simulink model "MultirotorSimPx4v1_8ContAttOnly"  (R2018b)
settings: Solver=VariableStepAuto  StartTime=0.0  StopTime=Simulation.T_END  MaxStep=Simulation.TS_MAX  RelTol=1e-3  EnableMultiTasking=on
PreLoadFcn:
  | % InitializeParameters;
undefined symbols (not defined in the file): Initial, Uav, Wind
libraries: simulink_extras x4, QuaternionLibrary x3
settings Model: Creator=jban039  LastModifiedBy=jban039
settings DataIOCC: Decimation=10  ExternalInput=getinputstruct(report10)  InitialState=getstatestruct(op)  LoadInitialState=on  SignalLogging=off  ReturnWorkspaceOutputs=on  OutputOption=SpecifiedOutputTimes  OutputTimes=Simulation.T_OUT
settings OptimizationCC: LifeSpan=inf
settings DebuggingCC: ReadBeforeWriteMsg=DisableAll  WriteAfterWriteMsg=DisableAll  WriteAfterReadMsg=DisableAll  MultiTaskDSMMsg=none  UnconnectedLineMsg=none  AllowSymbolicDim=off  SFUnexpectedBacktrackingDiag=warning  SFNoUnconditionalDefaultTransitionDiag=warning  SFExecutionAtInitializationDiag=none  UnderSpecifiedDimensionMsg=warning
settings ModelReferenceCC: UpdateModelReferenceTargets=IfOutOfDate  ModelReferenceMinAlgLoopOccurrences=on  PropagateSignalLabelsOutOfModel=off
settings SFSimCC: SFSimEcho=off  SimUseLocalCustomCode=off
settings RTWCC: RTWUseLocalCustomCode=off
settings CodeAppCC: StateflowObjectComments=on
settings GRTTargetCC: TargetLangStandard=C89/C90 (ANSI)
settings ConfigComp: CovMetricSettings=dw  CovHtmlReporting=on  CovSaveCumulativeToWorkspaceVar=on  CovSaveSingleToWorkspaceVar=on  CovExternalEMLEnable=off

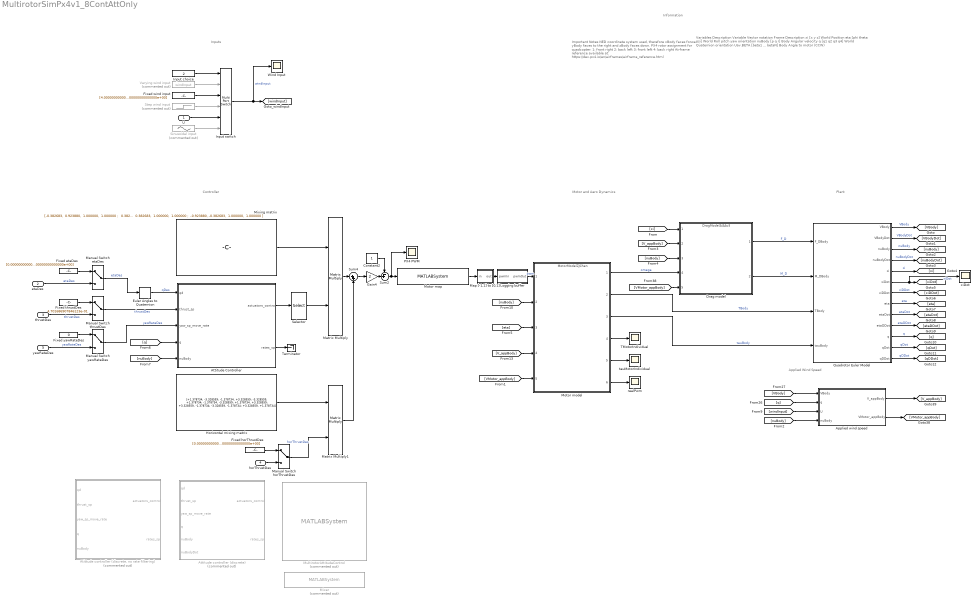
== system MultirotorSimPx4v1_8ContAttOnly ==
  note: Important Notes
      |
      | NED coordinate system used, therefore xBody faces forward, yBody faces to the right and zBody faces down.
      | PX4 rotor assignment for quadcopter:
      | 1: front right
      | 2: back left
      | 3: front left
      | 4: back right
      | Airframe reference available at:
      | https://dev.px4.io/en/airframes/airframe_reference.html
  note: Variables Description
      |
      | Variable
      | Vector notation
      | Frame
      | Description
      |
      | xi
      | [x y z]
      | World
      | Position
      |
      | eta
      | [phi theta psi]
      | World
      | Roll pitch yaw orientation
      |
      | nuBody
      | [p q r]
      | Body
      | Angular velocity
      |
      | q
      | [q1 q2 q3 q4]
      | World
      | Quaternion orientation
      |
      | Uav.BETA
      | [beta1 ... betaN]
      | Body
      | Angle to motor (CCW)
  note: Inputs
  note: Plant
  note: Motor and Aero Dynamics
  note: Information
  note: Controller
  note: Applied Wind Speed
  U : Inport  PortDimensions=3
  etaDes : Inport  Port=2  PortDimensions=[3,1]
  thrustDes : Inport  Port=3  PortDimensions=1
  horThrustDes : Inport  Port=4  PortDimensions=2
  yawRateDes : Inport  Port=5  PortDimensions=1
  Applied wind speed : Subsystem
  "Atittude controller (discrete, no rate filtering)" : Subsystem  Commented=on
  Attitude Controller : Subsystem
      mask Display: fprintf('MC_ATT_CONTROL\n\nCONTINUOUS')
  Attitude controller (discrete) : Subsystem  Commented=on
  Constant2 : Constant
  Drag model : ModelReference  ModelNameDialog=DragModelAIAAv3  SimulationMode=Normal  ModelReferenceVersion=1.368
  Euler Angles to Quaternion : QuaternionLibrary/Euler Angles to Quaternion
  Fixed etaDes : Constant  Value=[0.000000000000000e+00;-7.819550824259679e-02;0.000000000000000e+00]
  Fixed horThrustDes : Constant  Value=[0.000000000000000e+00;0.000000000000000e+00]
  Fixed thrustDes : Constant  Value=4.701686907846123e-01
  Fixed wind input : Constant  Value=[4.000000000000000e+00;0.000000000000000e+00;0.000000000000000e+00]
  Fixed yawRateDes : Constant  Value=0
  Gain4 : Gain  Gain=2
  Horizontal mixing matrix : Constant  Value=|
      | [+1.378734, -3.328559;
      |  -1.378734, +3.328559;
      |  -3.328559, +1.378734;
      |  -1.378734, -3.328559;
      |  +1.378734, +3.328559;
      |  +3.328559, -1.378734;
      |  -3.328559, -1.378734;
      |  +3.328559, +1.378734]
  Input choice : Constant  Value=2
  Input switch : MultiPortSwitch  Inputs=5
  Logging buffer : Subsystem
  Manual Switch etaDes : ManualSwitch
  Manual Switch horThrustDes : ManualSwitch
  Manual Switch thrustDes : ManualSwitch
  Manual Switch yawRateDes : ManualSwitch
  Map [-1,1] to [0,1] : Subsystem
  Matrix Multiply : Product  Multiplication=Matrix(*)
  Matrix Multiply1 : Product  Multiplication=Matrix(*)
  Mixer : MATLABSystem  Commented=on  SCDEnableBlockLinearizationSpecification=on  System=MultirotorMixer  airframeConfig=5  useHorThrust=0  outputSatStatus=0  SimulateUsing=Interpreted execution
      mask Type: MultirotorMixer
      mask Display:
      | disp(['MULTIROTOR' char(10) 'MIXER' char(10) 'octa_x']);
      | port_label('input',1,'actuatorsControl');
      | port_label('output',1,'px4PWM');
  Mixing matrix : Constant  Value=|
      | [-0.382683,  0.923880,  1.000000,  1.000000 ;
      |   0.382683, -0.923880,  1.000000,  1.000000 ;
      |  -0.923880,  0.382683, -1.000000,  1.000000 ;
      |  -0.382683, -0.923880, -1.000000,  1.000000 ;
      |   0.382683,  0.923880, -1.000000,  1.000000 ;
      |   0.923880, -0.382683, -1.000000,  1.000000 ;
      |   0.923880,  0.382683,  1.000000,  1.000000 ;
      |  -0.923880, -0.382683,  1.000000,  1.000000 ]
  Motor map : MATLABSystem  System=MotorMap  airframeConfig=5  SimulateUsing=Code generation
      mask Type: MotorMap
      mask Display:
      | disp(['MOTOR' char(10) 'MAP' char(10) 'octa_x']);
      | port_label('input',1,'px4PWM');
      | port_label('output',1,'simPWM');
  Motor model : ModelReference  ModelNameDialog=MotorModelZJChen  SimulationMode=Normal  ModelReferenceVersion=1.422
  MultirotorAttitudeControl : MATLABSystem  Commented=on  System=MulticopterAttitudeControl  acro_expo_rp=0.69  acro_expo_y=0.69  acro_pitch_max=720  acro_roll_max=720  acro_superexpo_rp=0.7  acro_superexpo_y=0.7  acro_yaw_max=540  airmode=0  d_term_cutoff_freq=30  pitch_rate_d=0.003  pitch_rate_ff=0  pitch_rate_i=0.05  pitch_rate_max=220  pitch_rate_p=0.15  pitch_p=6.5  pitch_rate_integ_lim=0.3  rattitude_thres=0.8  roll_rate_d=0.003  roll_rate_ff=0  roll_rate_i=0.05  roll_rate_max=220  roll_rate_p=0.15  roll_p=6.5  roll_rate_integ_lim=0.3  tpa_breakpoint_d=1  tpa_breakpoint_i=1  tpa_breakpoint_p=1  tpa_rate_d=0  tpa_rate_i=0  tpa_rate_p=0  yaw_rate_d=0  yaw_rate_ff=0  yaw_rate_i=0.1  yaw_rate_max=200  yaw_rate_p=0.2  yaw_auto_max=45  yaw_p=2.8  yaw_rate_integ_lim=0.3  man_throttle_min=0.08  man_tilt_max_deg=35  yaw_rate_scaling=200  throttle_hover=0.5  throttle_max=1  board_rotation_param=0  board_offset_x=0  board_offset_y=0  board_offset_z=0  bat_scale_en=0  throttle_curve=0  vehicle_status_is_rotary_wing=1  vehicle_status_is_vtol=0  loop_update_rate_hz=250  simple_mode=1  output_rates=0  SimulateUsing=Code generation
      mask Type: MulticopterAttitudeControl
      mask Display:
      | disp(['MulticopterAttitudeControl' char(10) '' char(10) 'v1.82']);
      | port_label('input',1,'qDes');
      | port_label('input',2,'thrustDes');
      | port_label('input',3,'yawRateDes');
      | port_label('input',4,'qMeasured');
      | port_label('input',5,'nuBody');
      | port_label('output',1,'actuatorsControl');
  PX4 PWM : Scope
  Quadrotor Euler Model : Subsystem
  Selector : Selector  InputPortWidth=8  IndexOptions=Index vector (dialog)  Indices=[1:4]  OutputSizes=1
  Sinusoidal input : Sin  Commented=on  Amplitude=Wind.Ampl  Bias=Wind.Bias  Frequency=Wind.Freq  SampleTime=0
  Step wind input : Step  Commented=on  Time=5  Before=[3 0 0]'  After=[5 0 0]'  SampleTime=0
  Sum2 : Sum  Inputs=-+|
  Sum4 : Sum  Inputs=|++
  TMotorIndividual : Scope
  Terminator : Terminator
  Varying wind input : FromWorkspace  Commented=on  VariableName=windInput  SampleTime=0
  Wind Input : Scope
  realPwm : Scope
  tauMotorIndividual : Scope
  xiDot : Scope
  wires:
  Motor model/1 -> Drag model/4  "omega"
  Motor model/2 -> Quadrotor Euler Model/3(TBody)  "TBody"
  Drag model/2 -> Quadrotor Euler Model/2(M_DBody)  "M_D"
  Quadrotor Euler Model/1(VBody) -> [VBody]  "VBody"
  Quadrotor Euler Model/2(VBodyDot) -> [VBodyDot]  "VBodyDot"
  Quadrotor Euler Model/3(nuBody) -> [nuBody]  "nuBody"
  Quadrotor Euler Model/4(nuBodyDot) -> [nuBodyDot]  "nuBodyDot"
  Quadrotor Euler Model/5(xi) -> [xi]  "xi"
  Quadrotor Euler Model/6(xiDot) -> xiDot/1, [xiDot]  "xiDot"
  Quadrotor Euler Model/7(xiDDot) -> [xiDDot]  "xiDDot"
  Quadrotor Euler Model/8(eta) -> [eta]  "eta"
  Quadrotor Euler Model/9(etaDot) -> [etaDot]  "etaDot"
  Quadrotor Euler Model/10(etaDDot) -> [etaDDot]  "etaDDot"
  [V_appBody] -> Drag model/2
  [nuBody] -> Motor model/2
  Quadrotor Euler Model/11(q) -> [q]  "q"
  Quadrotor Euler Model/12(qDot) -> [qDot]  "qDot"
  Quadrotor Euler Model/13(qDDot) -> [qDDot]  "qDDot"
  Drag model/1 -> Quadrotor Euler Model/1(F_DBody)  "F_D"
  Logging buffer/1(pwmOut) -> Motor model/1  "pwm"
  Sum2/1 -> PX4 PWM/1, Motor map/1
  [nuBody] -> Drag model/3
  [eta] -> Motor model/3
  [V_appBody] -> Motor model/4
  Motor model/4 -> TMotorIndividual/1
  Motor model/5 -> tauMotorIndividual/1
  [xi] -> Drag model/1
  [VMotor_appBody] -> Motor model/5
  [VMotor_appBody] -> Drag model/5
  Euler Angles to Quaternion/1 -> Attitude Controller/1(qd)  "qDes"
  Manual Switch thrustDes/1 -> Attitude Controller/2(thrust_sp)  "thrustDes"
  Manual Switch yawRateDes/1 -> Attitude Controller/3(yaw_sp_move_rate)  "yawRateDes"
  Motor model/3 -> Quadrotor Euler Model/4(tauBody)  "tauBody"
  [VBody] -> Applied wind speed/1(VBody)
  [q] -> Applied wind speed/2(q)
  [windInput] -> Applied wind speed/3(U)
  Applied wind speed/1(V_appBody) -> [V_appBody]
  Applied wind speed/2(VMotor_appBody) -> [VMotor_appBody]
  [nuBody] -> Applied wind speed/4(nuBody)
  Motor model/6 -> realPwm/1
  Motor map/1 -> Map [-1,1] to [0,1]/1(in)
  Map [-1,1] to [0,1]/1(out) -> Logging buffer/1(pwmIn)
  Selector/1 -> Matrix Multiply/2
  Manual Switch etaDes/1 -> Euler Angles to Quaternion/1  "etaDes"
  Attitude Controller/1(actuators_control) -> Selector/1
  Gain4/1 -> Sum2/2
  Constant2/1 -> Sum2/1
  Matrix Multiply/1 -> Sum4/1
  Matrix Multiply1/1 -> Sum4/2
  Manual Switch horThrustDes/1 -> Matrix Multiply1/2  "horThrustDes"
  Attitude Controller/2(rates_sp) -> Terminator/1
  Mixing matrix/1 -> Matrix Multiply/1
  Horizontal mixing matrix/1 -> Matrix Multiply1/1
  Sum4/1 -> Gain4/1
  [q] -> Attitude Controller/4(q)
  [nuBody] -> Attitude Controller/5(nuBody)
  Sinusoidal input/1 -> Input switch/6
  U/1 -> Input switch/5
  Input choice/1 -> Input switch/1
  Step wind input/1 -> Input switch/4
  Input switch/1 -> [windInput], Wind Input/1  "windInput"
  Fixed wind input/1 -> Input switch/3
  Varying wind input/1 -> Input switch/2
  Fixed horThrustDes/1 -> Manual Switch horThrustDes/1
  Fixed thrustDes/1 -> Manual Switch thrustDes/1
  Fixed etaDes/1 -> Manual Switch etaDes/1
  etaDes/1 -> Manual Switch etaDes/2  "etaDes"
  thrustDes/1 -> Manual Switch thrustDes/2  "thrustDes"
  yawRateDes/1 -> Manual Switch yawRateDes/2  "yawRateDes"
  horThrustDes/1 -> Manual Switch horThrustDes/2
  Fixed yawRateDes/1 -> Manual Switch yawRateDes/1

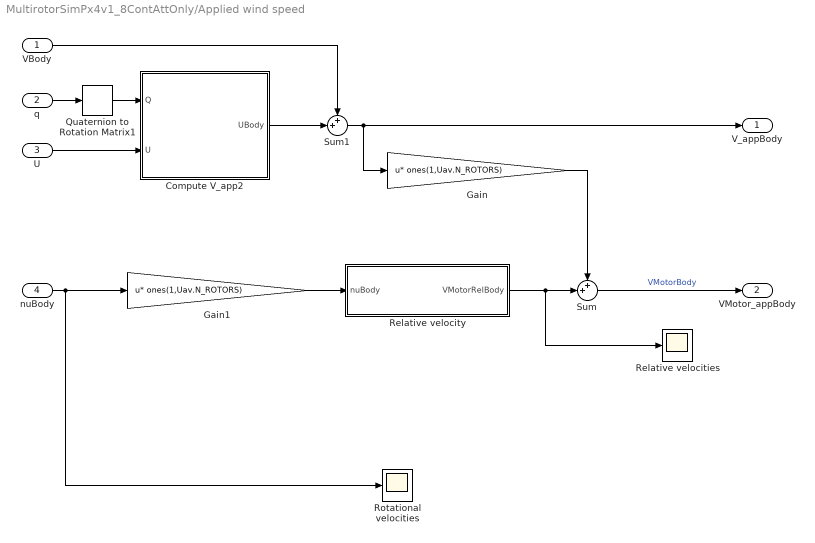
== system MultirotorSimPx4v1_8ContAttOnly/Applied wind speed ==
  VBody : Inport  Unit=m/s
  q : Inport  Port=2
  U : Inport  Port=3  Unit=m/s
  nuBody : Inport  Port=4  Unit=rad/s
  Compute V_app2 : MATLAB Function  TreatAsAtomicUnit=on
  Gain : Gain  Gain=ones(1,Uav.N_ROTORS)  Multiplication=Matrix(u*K)
  Gain1 : Gain  Gain=ones(1,Uav.N_ROTORS)  Multiplication=Matrix(u*K)
  Quaternion to Rotation Matrix1 : QuaternionLibrary/Quaternion to Rotation Matrix
  Relative velocities : Scope
  Relative velocity : MATLAB Function  TreatAsAtomicUnit=on
  Rotational velocities : Scope
  Sum : Sum  Inputs=++|
  Sum1 : Sum  Inputs=++|
  V_appBody : Outport  Unit=m/s
  VMotor_appBody : Outport  Port=2  Unit=m/s  PortDimensions=[3,Uav.N_ROTORS]
  wires:
  U/1 -> Compute V_app2/2(U)
  Sum/1 -> VMotor_appBody/1  "VMotorBody"
  Quaternion to Rotation Matrix1/1 -> Compute V_app2/1(Q)
  nuBody/1 -> Gain1/1, Rotational velocities/1
  Gain/1 -> Sum/1
  VBody/1 -> Sum1/1
  q/1 -> Quaternion to Rotation Matrix1/1
  Relative velocity/1(VMotorRelBody) -> Relative velocities/1, Sum/2
  Compute V_app2/1(UBody) -> Sum1/2
  Sum1/1 -> Gain/1, V_appBody/1
  Gain1/1 -> Relative velocity/1(nuBody)

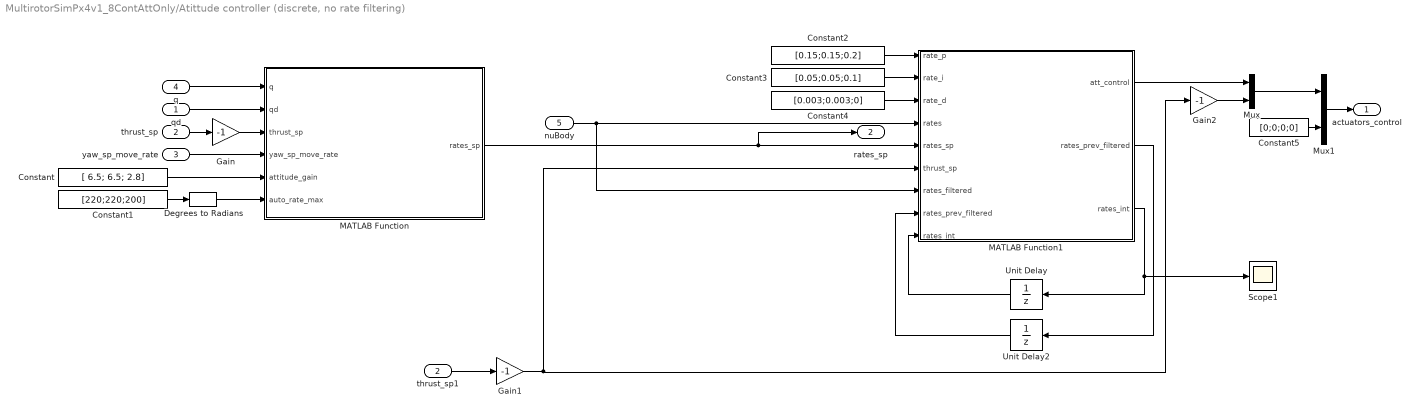
== system MultirotorSimPx4v1_8ContAttOnly/Atittude controller (discrete, no rate filtering) ==
  qd : Inport
  thrust_sp : Inport  Port=2
  yaw_sp_move_rate : Inport  Port=3
  q : Inport  Port=4
  nuBody : Inport  Port=5
  Constant : Constant  Value=[ 6.5; 6.5; 2.8]
  Constant1 : Constant  Value=[220;220;200]
  Constant2 : Constant  Value=[0.15;0.15;0.2]
  Constant3 : Constant  Value=[0.05;0.05;0.1]
  Constant4 : Constant  Value=[0.003;0.003;0]
  Constant5 : Constant  Value=[0;0;0;0]
  Degrees to Radians : simulink_extras/Transformations/Degrees to Radians
  Gain : Gain  Gain=-1
  Gain1 : Gain  Gain=-1
  Gain2 : Gain  Gain=-1
  MATLAB Function : MATLAB Function  TreatAsAtomicUnit=on  SystemSampleTime=1/250
  MATLAB Function1 : MATLAB Function  TreatAsAtomicUnit=on  SystemSampleTime=1/250
  Mux : Mux  Inputs=2
  Mux1 : Mux  Inputs=2
  Scope1 : Scope
  Unit Delay : UnitDelay  SampleTime=1/250  StateName=rates_int
  Unit Delay2 : UnitDelay  SampleTime=1/250  StateName=rates_prev_filtered
  thrust_sp1 : InportShadow  Port=2
  actuators_control : Outport
  rates_sp : Outport  Port=2
  wires:
  qd/1 -> MATLAB Function/2(qd)
  q/1 -> MATLAB Function/1(q)
  Constant/1 -> MATLAB Function/5(attitude_gain)
  Constant1/1 -> Degrees to Radians/1
  Degrees to Radians/1 -> MATLAB Function/6(auto_rate_max)
  yaw_sp_move_rate/1 -> MATLAB Function/4(yaw_sp_move_rate)
  Constant4/1 -> MATLAB Function1/3(rate_d)
  Constant3/1 -> MATLAB Function1/2(rate_i)
  Constant2/1 -> MATLAB Function1/1(rate_p)
  MATLAB Function1/1(att_control) -> Mux/1
  nuBody/1 -> MATLAB Function1/7(rates_filtered), MATLAB Function1/4(rates)
  Unit Delay/1 -> MATLAB Function1/9("rates_int ")
  MATLAB Function1/3(rates_int) -> Unit Delay/1, Scope1/1
  Mux/1 -> Mux1/1
  Unit Delay2/1 -> MATLAB Function1/8("rates_prev_filtered ")
  MATLAB Function1/2(rates_prev_filtered) -> Unit Delay2/1
  thrust_sp1/1 -> Gain1/1
  Constant5/1 -> Mux1/2
  Mux1/1 -> actuators_control/1
  thrust_sp/1 -> Gain/1
  MATLAB Function/1(rates_sp) -> MATLAB Function1/5(rates_sp), rates_sp/1
  Gain/1 -> MATLAB Function/3(thrust_sp)
  Gain1/1 -> Gain2/1, MATLAB Function1/6(thrust_sp)
  Gain2/1 -> Mux/2

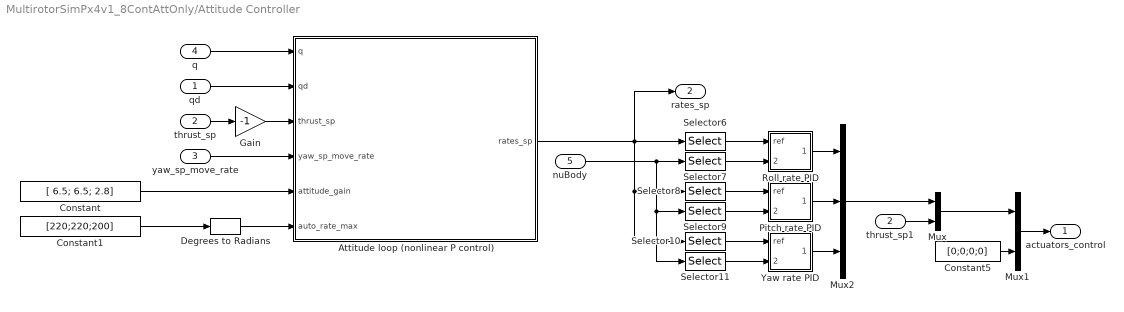
== system MultirotorSimPx4v1_8ContAttOnly/Attitude Controller ==
  qd : Inport
  thrust_sp : Inport  Port=2  PortDimensions=1
  yaw_sp_move_rate : Inport  Port=3
  q : Inport  Port=4
  nuBody : Inport  Port=5
  Attitude loop (nonlinear P control) : MATLAB Function  TreatAsAtomicUnit=on
  Constant : Constant  Value=[ 6.5; 6.5; 2.8]
  Constant1 : Constant  Value=[220;220;200]
  Constant5 : Constant  Value=[0;0;0;0]
  Degrees to Radians : simulink_extras/Transformations/Degrees to Radians
  Gain : Gain  Gain=-1
  Mux : Mux  Inputs=2
  Mux1 : Mux  Inputs=2
  Mux2 : Mux  Inputs=3
  Pitch rate PID : Subsystem  mask{PID_P=0.15, PID_I=0.05, PID_D=0.003, PID_FC=30, PID_I_STATENAME='AttRatePID_I_pitch', PID_D_STATENAME='AttRatePID_D_pitch'}
      mask prompts: PID_P "P gain"; PID_I "I gain"; PID_D "D gain"; PID_FC "D filter cutoff (Hz)"; PID_I_STATENAME "Integartor state name"; PID_D_STATENAME "D filter state name"
      mask DialogControl DescGroupVar Prompt: PID Controller with Second Order Derivative Filter
      mask DialogControl DescTextVar Prompt: The derivative gain is applied on the derivative of y rather than that of the error (r-y).
      mask Display:
      | disp('PID(s)')
      | port_label('input', 1, 'r')
      | port_label('input', 2, 'y')
      | text(1,0,'2^{nd}','horizontalAlignment','right','interpreter','tex','verticalAlignment','bottom')
  Roll rate PID : Subsystem  mask{PID_P=0.15, PID_I=0.05, PID_D=0.003, PID_FC=30, PID_I_STATENAME='AttRatePID_I_roll', PID_D_STATENAME='AttRatePID_D_roll'}
      mask prompts: PID_P "P gain"; PID_I "I gain"; PID_D "D gain"; PID_FC "D filter cutoff (Hz)"; PID_I_STATENAME "Integartor state name"; PID_D_STATENAME "D filter state name"
      mask DialogControl DescGroupVar Prompt: PID Controller with Second Order Derivative Filter
      mask DialogControl DescTextVar Prompt: The derivative gain is applied on the derivative of y rather than that of the error (r-y).
      mask Display:
      | disp('PID(s)')
      | port_label('input', 1, 'r')
      | port_label('input', 2, 'y')
      | text(1,0,'2^{nd}','horizontalAlignment','right','interpreter','tex','verticalAlignment','bottom')
  Selector10 : Selector  InputPortWidth=3  IndexOptions=Index vector (dialog)  Indices=3  OutputSizes=1
  Selector11 : Selector  InputPortWidth=3  IndexOptions=Index vector (dialog)  Indices=3  OutputSizes=1
  Selector6 : Selector  InputPortWidth=3  IndexOptions=Index vector (dialog)  Indices=1  OutputSizes=1
  Selector7 : Selector  InputPortWidth=3  IndexOptions=Index vector (dialog)  Indices=1  OutputSizes=1
  Selector8 : Selector  InputPortWidth=3  IndexOptions=Index vector (dialog)  Indices=2  OutputSizes=1
  Selector9 : Selector  InputPortWidth=3  IndexOptions=Index vector (dialog)  Indices=2  OutputSizes=1
  Yaw rate PID : Subsystem  mask{PID_P=0.2, PID_I=0.1, PID_D=0, PID_FC=30, PID_I_STATENAME='AttRatePID_I_yaw', PID_D_STATENAME='AttRatePID_D_yaw'}
      mask prompts: PID_P "P gain"; PID_I "I gain"; PID_D "D gain"; PID_FC "D filter cutoff (Hz)"; PID_I_STATENAME "Integartor state name"; PID_D_STATENAME "D filter state name"
      mask DialogControl DescGroupVar Prompt: PID Controller with Second Order Derivative Filter
      mask DialogControl DescTextVar Prompt: The derivative gain is applied on the derivative of y rather than that of the error (r-y).
      mask Display:
      | disp('PID(s)')
      | port_label('input', 1, 'r')
      | port_label('input', 2, 'y')
      | text(1,0,'2^{nd}','horizontalAlignment','right','interpreter','tex','verticalAlignment','bottom')
  thrust_sp1 : InportShadow  Port=2  PortDimensions=1
  actuators_control : Outport  PortDimensions=8
  rates_sp : Outport  Port=2
  wires:
  nuBody/1 -> Selector7/1, Selector9/1, Selector11/1
  Selector9/1 -> Pitch rate PID/2(meas)
  Selector11/1 -> Yaw rate PID/2(meas)
  Selector10/1 -> Yaw rate PID/1(ref)
  Selector8/1 -> Pitch rate PID/1(ref)
  Selector7/1 -> Roll rate PID/2(meas)
  Selector6/1 -> Roll rate PID/1(ref)
  Mux2/1 -> Mux/1
  Pitch rate PID/1(Out) -> Mux2/2
  Roll rate PID/1(Out) -> Mux2/1
  Yaw rate PID/1(Out) -> Mux2/3
  qd/1 -> Attitude loop (nonlinear P control)/2(qd)
  q/1 -> Attitude loop (nonlinear P control)/1(q)
  Constant/1 -> Attitude loop (nonlinear P control)/5(attitude_gain)
  Constant1/1 -> Degrees to Radians/1
  Degrees to Radians/1 -> Attitude loop (nonlinear P control)/6(auto_rate_max)
  yaw_sp_move_rate/1 -> Attitude loop (nonlinear P control)/4(yaw_sp_move_rate)
  Mux/1 -> Mux1/1
  Constant5/1 -> Mux1/2
  Mux1/1 -> actuators_control/1
  thrust_sp/1 -> Gain/1
  Attitude loop (nonlinear P control)/1(rates_sp) -> Selector6/1, Selector8/1, Selector10/1, rates_sp/1
  Gain/1 -> Attitude loop (nonlinear P control)/3(thrust_sp)
  thrust_sp1/1 -> Mux/2

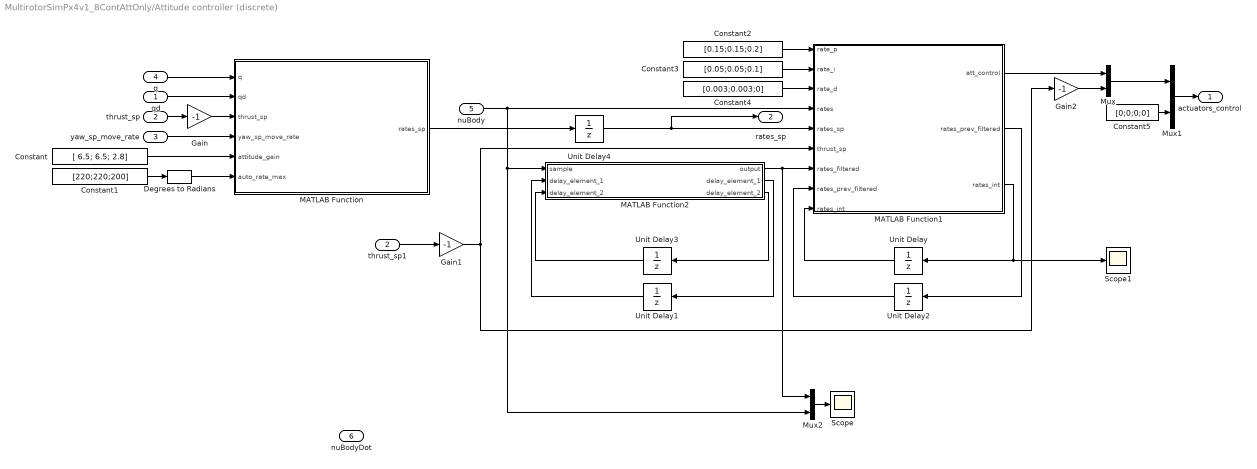
== system MultirotorSimPx4v1_8ContAttOnly/Attitude controller (discrete) ==
  qd : Inport
  thrust_sp : Inport  Port=2
  yaw_sp_move_rate : Inport  Port=3
  q : Inport  Port=4
  nuBody : Inport  Port=5
  nuBodyDot : Inport  Port=6
  Constant : Constant  Value=[ 6.5; 6.5; 2.8]
  Constant1 : Constant  Value=[220;220;200]
  Constant2 : Constant  Value=[0.15;0.15;0.2]
  Constant3 : Constant  Value=[0.05;0.05;0.1]
  Constant4 : Constant  Value=[0.003;0.003;0]
  Constant5 : Constant  Value=[0;0;0;0]
  Degrees to Radians : simulink_extras/Transformations/Degrees to Radians
  Gain : Gain  Gain=-1
  Gain1 : Gain  Gain=-1
  Gain2 : Gain  Gain=-1
  MATLAB Function : MATLAB Function  TreatAsAtomicUnit=on  SystemSampleTime=1/250
  MATLAB Function1 : MATLAB Function  TreatAsAtomicUnit=on  SystemSampleTime=1/250
  MATLAB Function2 : MATLAB Function  TreatAsAtomicUnit=on  SystemSampleTime=1/250
  Mux : Mux  Inputs=2
  Mux1 : Mux  Inputs=2
  Mux2 : Mux  Inputs=2
  Scope : Scope
  Scope1 : Scope
  Unit Delay : UnitDelay  SampleTime=1/250  StateName=rates_int
  Unit Delay1 : UnitDelay  SampleTime=1/250  StateName=lp_filters_d_delay_element_1
  Unit Delay2 : UnitDelay  SampleTime=1/250  StateName=rates_prev_filtered
  Unit Delay3 : UnitDelay  SampleTime=1/250  StateName=lp_filters_d_delay_element_2
  Unit Delay4 : UnitDelay  SampleTime=1/250  StateName=rates_sp
  thrust_sp1 : InportShadow  Port=2
  actuators_control : Outport
  rates_sp : Outport  Port=2
  wires:
  qd/1 -> MATLAB Function/2(qd)
  q/1 -> MATLAB Function/1(q)
  Constant/1 -> MATLAB Function/5(attitude_gain)
  Constant1/1 -> Degrees to Radians/1
  Degrees to Radians/1 -> MATLAB Function/6(auto_rate_max)
  yaw_sp_move_rate/1 -> MATLAB Function/4(yaw_sp_move_rate)
  Constant4/1 -> MATLAB Function1/3(rate_d)
  Constant3/1 -> MATLAB Function1/2(rate_i)
  Constant2/1 -> MATLAB Function1/1(rate_p)
  MATLAB Function/1(rates_sp) -> Unit Delay4/1
  MATLAB Function1/1(att_control) -> Mux/1
  nuBody/1 -> MATLAB Function1/4(rates), MATLAB Function2/1(sample), Mux2/2
  Unit Delay/1 -> MATLAB Function1/9("rates_int ")
  MATLAB Function1/3(rates_int) -> Unit Delay/1, Scope1/1
  Unit Delay1/1 -> MATLAB Function2/2("delay_element_1 ")
  Mux/1 -> Mux1/1
  Unit Delay2/1 -> MATLAB Function1/8("rates_prev_filtered ")
  MATLAB Function1/2(rates_prev_filtered) -> Unit Delay2/1
  Unit Delay3/1 -> MATLAB Function2/3("delay_element_2 ")
  MATLAB Function2/3(delay_element_2) -> Unit Delay3/1
  MATLAB Function2/2(delay_element_1) -> Unit Delay1/1
  thrust_sp1/1 -> Gain1/1
  Constant5/1 -> Mux1/2
  Mux1/1 -> actuators_control/1
  thrust_sp/1 -> Gain/1
  Mux2/1 -> Scope/1
  Unit Delay4/1 -> MATLAB Function1/5(rates_sp), rates_sp/1
  Gain/1 -> MATLAB Function/3(thrust_sp)
  Gain1/1 -> Gain2/1, MATLAB Function1/6(thrust_sp)
  Gain2/1 -> Mux/2
  MATLAB Function2/1(output) -> Mux2/1, MATLAB Function1/7(rates_filtered)

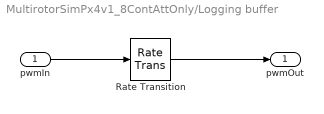
== system MultirotorSimPx4v1_8ContAttOnly/Logging buffer ==
  pwmIn : Inport
  Rate Transition : RateTransition  SCDEnableBlockLinearizationSpecification=on
  pwmOut : Outport
  wires:
  pwmIn/1 -> Rate Transition/1
  Rate Transition/1 -> pwmOut/1

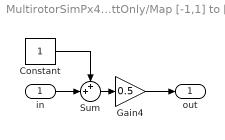
== system MultirotorSimPx4v1_8ContAttOnly/Map [-1,1] to [0,1] ==
  in : Inport
  Constant : Constant
  Gain4 : Gain  Gain=0.5
  Sum : Sum  Inputs=++|
  out : Outport
  wires:
  Sum/1 -> Gain4/1
  Gain4/1 -> out/1
  in/1 -> Sum/2
  Constant/1 -> Sum/1

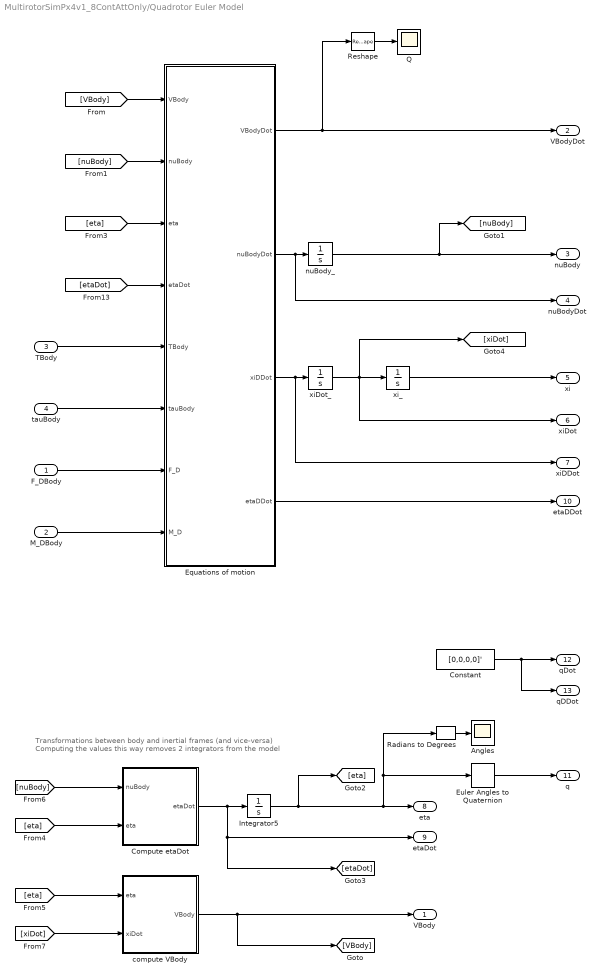
== system MultirotorSimPx4v1_8ContAttOnly/Quadrotor Euler Model ==
  note: Transformations between body and inertial frames (and vice-versa)
      | Computing the values this way removes 2 integrators from the model
  F_DBody : Inport  Unit=N
  M_DBody : Inport  Port=2  Unit=N*m
  TBody : Inport  Port=3  Unit=N
  tauBody : Inport  Port=4  Unit=N*m
  Angles : Scope
  Compute etaDot : MATLAB Function  TreatAsAtomicUnit=on
  Constant : Constant  Value=[0,0,0,0]'
  Equations of motion : MATLAB Function  TreatAsAtomicUnit=on
  Euler Angles to Quaternion : QuaternionLibrary/Euler Angles to Quaternion
  Integrator5 : Integrator  InitialCondition=Initial.ETA  ContinuousStateAttributes='eta'
  Q : Scope
  Radians to Degrees : simulink_extras/Transformations/Radians to Degrees
  Reshape : Reshape  OutputDimensionality=Column vector (2-D)
  compute VBody : MATLAB Function  TreatAsAtomicUnit=on
  nuBody_ : Integrator  InitialCondition=Initial.NU_BODY  ContinuousStateAttributes='nuBody'
  xiDot_ : Integrator  InitialCondition=Initial.XI_DOT  ContinuousStateAttributes='xiDot'
  xi_ : Integrator  InitialCondition=Initial.XI  ContinuousStateAttributes='xi'
  VBody : Outport  Unit=m/s
  VBodyDot : Outport  Port=2  Unit=m/s^2
  nuBody : Outport  Port=3  Unit=rad/s
  nuBodyDot : Outport  Port=4  Unit=rad/s^2
  xi : Outport  Port=5  Unit=m
  xiDot : Outport  Port=6  Unit=m/s
  xiDDot : Outport  Port=7  Unit=m/s^2
  eta : Outport  Port=8  Unit=rad
  etaDot : Outport  Port=9  Unit=rad/s
  etaDDot : Outport  Port=10  Unit=rad/s^2
  q : Outport  Port=11
  qDot : Outport  Port=12
  qDDot : Outport  Port=13
  wires:
  Radians to Degrees/1 -> Angles/1
  Constant/1 -> qDot/1, qDDot/1
  Euler Angles to Quaternion/1 -> q/1
  Integrator5/1 -> [eta], eta/1, Euler Angles to Quaternion/1, Radians to Degrees/1
  Compute etaDot/1(etaDot) -> Integrator5/1, [etaDot], etaDot/1
  [eta] -> Compute etaDot/2(eta)
  compute VBody/1(VBody) -> [VBody], VBody/1
  [eta] -> compute VBody/1(eta)
  [nuBody] -> Compute etaDot/1(nuBody)
  [xiDot] -> compute VBody/2(xiDot)
  [etaDot] -> Equations of motion/4(etaDot)
  xiDot_/1 -> xiDot/1, [xiDot], xi_/1
  Reshape/1 -> Q/1
  Equations of motion/4(etaDDot) -> etaDDot/1
  [eta] -> Equations of motion/3(eta)
  Equations of motion/2(nuBodyDot) -> nuBodyDot/1, nuBody_/1
  nuBody_/1 -> nuBody/1, [nuBody]
  M_DBody/1 -> Equations of motion/8(M_D)
  F_DBody/1 -> Equations of motion/7(F_D)
  Equations of motion/3(xiDDot) -> xiDDot/1, xiDot_/1
  TBody/1 -> Equations of motion/5(TBody)
  tauBody/1 -> Equations of motion/6(tauBody)
  [VBody] -> Equations of motion/1(VBody)
  [nuBody] -> Equations of motion/2(nuBody)
  xi_/1 -> xi/1
  Equations of motion/1(VBodyDot) -> VBodyDot/1, Reshape/1

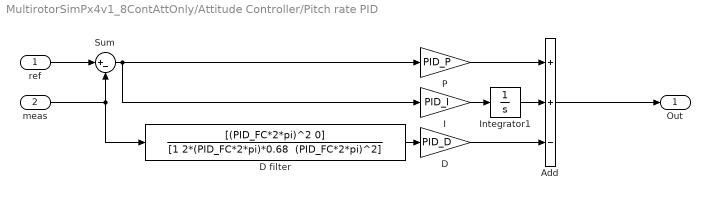
== system MultirotorSimPx4v1_8ContAttOnly/Attitude Controller/Pitch rate PID ==
  ref : Inport
  meas : Inport  Port=2
  Add : Sum  Inputs=++-
  D : Gain  Gain=PID_D
  D filter : TransferFcn  Numerator=[(PID_FC*2*pi)^2 0]  Denominator="[1 2*(PID_FC*2*pi)*0.68  (PID_FC*2*pi)^2]"  ContinuousStateAttributes=PID_D_STATENAME
  I : Gain  Gain=PID_I
  Integrator1 : Integrator  LimitOutput=on  UpperSaturationLimit=0.3  LowerSaturationLimit=-0.3  ContinuousStateAttributes=PID_I_STATENAME
  P : Gain  Gain=PID_P
  Sum : Sum  Inputs=|+-
  Out : Outport
  wires:
  Add/1 -> Out/1
  P/1 -> Add/1
  Integrator1/1 -> Add/2
  D filter/1 -> D/1
  Sum/1 -> P/1, I/1
  D/1 -> Add/3
  I/1 -> Integrator1/1
  ref/1 -> Sum/1
  meas/1 -> D filter/1, Sum/2

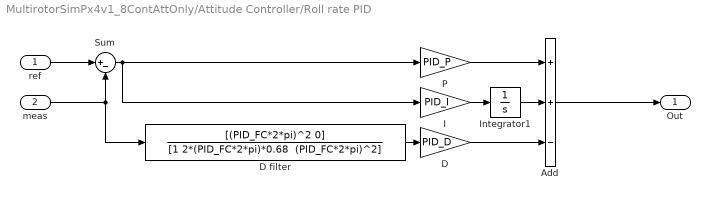
== system MultirotorSimPx4v1_8ContAttOnly/Attitude Controller/Roll rate PID ==
  ref : Inport
  meas : Inport  Port=2
  Add : Sum  Inputs=++-
  D : Gain  Gain=PID_D
  D filter : TransferFcn  Numerator=[(PID_FC*2*pi)^2 0]  Denominator="[1 2*(PID_FC*2*pi)*0.68  (PID_FC*2*pi)^2]"  ContinuousStateAttributes=PID_D_STATENAME
  I : Gain  Gain=PID_I
  Integrator1 : Integrator  LimitOutput=on  UpperSaturationLimit=0.3  LowerSaturationLimit=-0.3  ContinuousStateAttributes=PID_I_STATENAME
  P : Gain  Gain=PID_P
  Sum : Sum  Inputs=|+-
  Out : Outport
  wires:
  meas/1 -> Sum/2, D filter/1
  ref/1 -> Sum/1
  I/1 -> Integrator1/1
  D/1 -> Add/3
  Sum/1 -> I/1, P/1
  D filter/1 -> D/1
  Integrator1/1 -> Add/2
  P/1 -> Add/1
  Add/1 -> Out/1

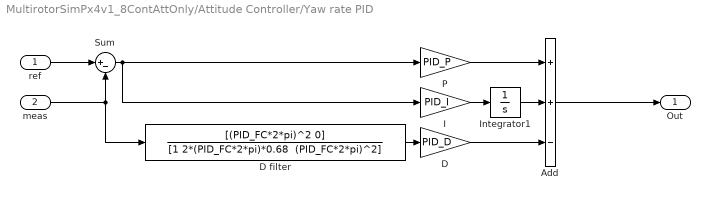
== system MultirotorSimPx4v1_8ContAttOnly/Attitude Controller/Yaw rate PID ==
  ref : Inport
  meas : Inport  Port=2
  Add : Sum  Inputs=++-
  D : Gain  Gain=PID_D
  D filter : TransferFcn  Numerator=[(PID_FC*2*pi)^2 0]  Denominator="[1 2*(PID_FC*2*pi)*0.68  (PID_FC*2*pi)^2]"  ContinuousStateAttributes=PID_D_STATENAME
  I : Gain  Gain=PID_I
  Integrator1 : Integrator  LimitOutput=on  UpperSaturationLimit=0.3  LowerSaturationLimit=-0.3  ContinuousStateAttributes=PID_I_STATENAME
  P : Gain  Gain=PID_P
  Sum : Sum  Inputs=|+-
  Out : Outport
  wires:
  meas/1 -> Sum/2, D filter/1
  ref/1 -> Sum/1
  I/1 -> Integrator1/1
  D/1 -> Add/3
  Sum/1 -> I/1, P/1
  D filter/1 -> D/1
  Integrator1/1 -> Add/2
  P/1 -> Add/1
  Add/1 -> Out/1

== matlab function MultirotorSimPx4v1_8ContAttOnly/Quadrotor Euler Model/Equations of motion ==
  data: VBody input; VBodyDot output; nuBody input; eta input; etaDot input; TBody input size=3; tauBody input size=3; F_D input size=3; M_D input size=3; nuBodyDot output; Uav parameter; xiDDot output; etaDDot output
function [VBodyDot, nuBodyDot, xiDDot, etaDDot] = QuadrotorQuaternionModel(...
    VBody, nuBody, eta, etaDot, TBody, tauBody, F_D, M_D, Uav )
%#codegen

%% Rotation matrices
% Precompute sines and cosines
sPhi   = sin(eta(1));
sTheta = sin(eta(2));
sPsi   = sin(eta(3));
cPhi   = cos(eta(1));
cTheta = cos(eta(2));
cPsi   = cos(eta(3));
tTheta = tan(eta(2));

phiDot   = etaDot(1);
thetaDot = etaDot(2);

% Body frame to inertial frame
R = [cPsi*cTheta, cPsi*sTheta*sPhi-sPsi*cPhi, cPsi*sTheta*cPhi+sPsi*sPhi;
     sPsi*cTheta, sPsi*sTheta*sPhi+cPsi*cPhi, sPsi*sTheta*cPhi-cPsi*sPhi;
     -sTheta,     cTheta*sPhi,                cTheta*cPhi+sPsi*sPhi];

WInvertDot = [...
    0,  phiDot*cPhi*tTheta+thetaDot*sPhi/cTheta^2,    -phiDot*sPhi*cTheta+thetaDot*cPhi/cTheta^2;
    0, -phiDot*sPhi,                                  -phiDot*cPhi;
	0,  phiDot*cPhi/cTheta+phiDot*sPhi*tTheta/cTheta, -phiDot*sPhi/cTheta+thetaDot*cPhi*tTheta/cTheta];

WInvert = [1, sPhi*tTheta,  cPhi*tTheta;
           0, cPhi,        -sPhi;
           0, sPhi/cTheta,  cPhi/cTheta];


%% Moments and Forces
% Body frame accelerations
VBodyDot  = (1/Uav.M) * (R'*Uav.G + TBody - cross(nuBody, Uav.M*VBody) + F_D);
nuBodyDot = Uav.I \ (tauBody - cross(nuBody, Uav.I*nuBody) + M_D);

% Inertial frame accelerations
xiDDot = (1/Uav.M)*(Uav.G + R*TBody + R*F_D);
etaDDot = WInvertDot*nuBody + WInvert*nuBodyDot;

end

== matlab function MultirotorSimPx4v1_8ContAttOnly/Atittude controller (discrete, no rate filtering)/MATLAB Function ==
  data: q input; rates_sp output; qd input; thrust_sp input; yaw_sp_move_rate input; attitude_gain input; auto_rate_max input
function rates_sp  = control_attitude( q, qd, thrust_sp, ...
    yaw_sp_move_rate, attitude_gain, auto_rate_max )

%thrust_sp = -thrust_sp;

roll_pitch_gain = ( attitude_gain(1) + attitude_gain(2) ) / 2;
yaw_w = constrain( attitude_gain(3) / roll_pitch_gain, 0, 1 );
attitude_gain(3) = roll_pitch_gain;

q  = q  ./ norm(q);
qd = qd ./ norm(qd);

e_z   = QuatToDcmZ( q );
e_z_d = QuatToDcmZ( qd );
qd_red = VecsToQuat( e_z, e_z_d );

qd_red = QuatMult( qd_red, q );

q_mix = QuatMult( InvertQuat(qd_red), qd );
q_mix = q_mix .* SignNoZero( q_mix(1) );

q_mix(1) = constrain( q_mix(1), -1, 1 );
q_mix(4) = constrain( q_mix(4), -1, 1 );
qd = QuatMult( qd_red, ...
    [ cos( yaw_w * acos(q_mix(1)) );
    0;
    0;
    sin( yaw_w * asin(q_mix(4)) ) ] );

qe = QuatMult( InvertQuat(q), qd );

eq = 2 .* SignNoZero(qe(1)) .* qe(2:4);

rates_sp = eq .* attitude_gain;

rates_sp = rates_sp + QuatToDcmZ( InvertQuat(q) ) .* yaw_sp_move_rate;

rates_sp = constrain( rates_sp, -auto_rate_max, auto_rate_max);
end

function y = constrain( x, x_min, x_max )
    y = max( min(x, x_max), x_min );
end

function dcmZ = QuatToDcmZ( quat )
    a = quat(1);
    b = quat(2);
    c = quat(3);
    d = quat(4);
    dcmZ = [ 2 * (a * c + b * d);
        2 * (c * d - a * b);
        a * a - b * b - c * c + d * d ];
end

function quat = VecsToQuat( src, dst )
    cr = cross(src, dst);
    dt = dot(src, dst);
    quat = zeros(4,1);
    locEps = 1e-5; % Don't use eps as it's a reserved variable in MATLAB
    if (norm(cr) < locEps && dt < 0)
        % Handle corner cases with 180 degree rotations
        % If the two vectors are parallel, cross product is zero
        % If they point opposite, the dot product is negative
        cr = abs(src);
        if (cr(1) < cr(2))
            if (cr(1) < cr(3))
                cr = [1; 0; 0];
            else
                cr = [0; 0; 1];
            end
        else
            if (cr(2) < cr(3))
                cr = [0; 1; 0];
            else
                cr = [0; 0; 1];
            end
        end
        quat(1) = 0;
        cr = cross(src, cr);
    else
        % Normal case, do half-way quaternion solution
        quat(1) = dt + sqrt( norm(src)^2 * norm(dst)^2 );
    end
    quat(2) = cr(1);
    quat(3) = cr(2);
    quat(4) = cr(3);
    quat = MulticopterAttitudeControl.normalize( quat );
end

function quatInv = InvertQuat( quat )
    normSq = dot( quat, quat );
    quatInv = ( quat .* [1;-1;-1;-1] ./ normSq );
end

function quatOut = QuatMult( q1, q2 )
    quatOut = [ q1(1) * q2(1) - q1(2) * q2(2) - q1(3) * q2(3) - q1(4) * q2(4) ;
        q1(1) * q2(2) + q1(2) * q2(1) + q1(3) * q2(4) - q1(4) * q2(3) ;
        q1(1) * q2(3) - q1(2) * q2(4) + q1(3) * q2(1) + q1(4) * q2(2) ;
        q1(1) * q2(4) + q1(2) * q2(3) - q1(3) * q2(2) + q1(4) * q2(1) ];
end

function out = SignNoZero( in )
    out = ( 0 <= in ) - ( in < 0 );
end

== matlab function MultirotorSimPx4v1_8ContAttOnly/Atittude controller (discrete, no rate filtering)/MATLAB Function1 ==
  data: rate_p input; rate_i input; rate_d input; rates input; att_control output; rates_prev_filtered output; rates_sp input size=3; thrust_sp input; rates_filtered input size=3; rates_prev_filtered input size=3; rates_int output; rates_int input size=3
function [att_control, rates_prev_filtered, rates_int] = control_attitude_rates( rate_p, rate_i, rate_d, ...
    rates, rates_sp, thrust_sp, rates_filtered, rates_prev_filtered, rates_int )

    % values
    rate_int_lim = [ 0.3; 0.3; 0.3 ];
    tpa_breakpoint_p = 1;
    tpa_breakpoint_i = 1;
    tpa_breakpoint_d = 1;
    tpa_rate_p = 0;
    tpa_rate_i = 0;
    tpa_rate_d = 0;
    dt = 1/250;
    rate_ff = zeros(3,1);
    
    rates_p_scaled = rate_p .* pid_attenuations( tpa_breakpoint_p, tpa_rate_p, thrust_sp );
    rates_i_scaled = rate_i .* pid_attenuations( tpa_breakpoint_i, tpa_rate_i, thrust_sp );
    rates_d_scaled = rate_d .* pid_attenuations( tpa_breakpoint_d, tpa_rate_d, thrust_sp );

    rates_err = rates_sp - rates;

    %rates_filtered = LowPassFilter2pVector3Apply( obj, rates );

    att_control = rates_p_scaled .* rates_err + ...
        rates_int - ...
        rates_d_scaled .* (rates_filtered - rates_prev_filtered) / dt + ...
        rate_ff .* rates_sp;

    rates_prev_filtered = rates_filtered;

    rate_i_tmp = rates_int + rates_i_scaled .* rates_err .* dt;
    
    toKeep = isfinite(rate_i_tmp) & (rate_i_tmp > -rate_int_lim) & ...
                (rate_i_tmp < rate_int_lim);
    %rates_int = zeros(3,1);
    rates_int(toKeep) = rate_i_tmp(toKeep);
    
    rates_int = constrain( rates_int, -rate_int_lim, rate_int_lim );
end

function pidAttenuationPerAxis = pid_attenuations( tpa_breakpoint, tpa_rate, thrust_sp )
    TPA_RATE_LOWER_LIMIT = 0.05;
    tpa = 1.0 - tpa_rate * (abs(thrust_sp) - tpa_breakpoint) / (1.0 - tpa_breakpoint);
    tpa = max([TPA_RATE_LOWER_LIMIT, min([1.0, tpa])]);
    pidAttenuationPerAxis = [ tpa; tpa; 1.0 ];
end

function y = constrain( x, x_min, x_max )
    y = max( min(x, x_max), x_min );
end

== matlab function MultirotorSimPx4v1_8ContAttOnly/Applied wind speed/Relative velocity ==
  data: nuBody input; Uav parameter; VMotorRelBody output
function VMotorRelBody = relativeMotorVelocity( nuBody , Uav )
%#codegen
    VMotorRelBody = cross( nuBody, Uav.L_VEC );
end

== matlab function MultirotorSimPx4v1_8ContAttOnly/Applied wind speed/Compute V_app2 ==
  data: Q input; UBody output; U input size=3
function UBody = computeUBody(Q, U)
%#codegen

% Rotation matrix from Wind frame to Inertial frame
% Wind frame SEU, inertial frame NED
R_U = [1,  0, 0;
       0, -1, 0;
       0,  0, 1];
   
UBody = Q' * R_U * U;

== matlab function MultirotorSimPx4v1_8ContAttOnly/Attitude Controller/Attitude loop (nonlinear P control) ==
  data: q input; rates_sp output; qd input; thrust_sp input; yaw_sp_move_rate input; attitude_gain input; auto_rate_max input
function rates_sp  = control_attitude( q, qd, thrust_sp, ...
    yaw_sp_move_rate, attitude_gain, auto_rate_max )
    %thrust_sp = -thrust_sp;

    roll_pitch_gain = ( attitude_gain(1) + attitude_gain(2) ) / 2;
    yaw_w = constrain( attitude_gain(3) / roll_pitch_gain, 0, 1 );
    attitude_gain(3) = roll_pitch_gain;

    q  = q  ./ norm(q);
    qd = qd ./ norm(qd);

    e_z   = QuatToDcmZ( q );
    e_z_d = QuatToDcmZ( qd );
    qd_red = VecsToQuat( e_z, e_z_d );

    qd_red = QuatMult( qd_red, q );

    q_mix = QuatMult( InvertQuat(qd_red), qd );
    q_mix = q_mix .* SignNoZero( q_mix(1) );

    q_mix(1) = constrain( q_mix(1), -1, 1 );
    q_mix(4) = constrain( q_mix(4), -1, 1 );
    qd = QuatMult( qd_red, ...
        [ cos( yaw_w * acos(q_mix(1)) );
        0;
        0;
        sin( yaw_w * asin(q_mix(4)) ) ] );

    qe = QuatMult( InvertQuat(q), qd );

    eq = 2 .* SignNoZero(qe(1)) .* qe(2:4);

    rates_sp = eq .* attitude_gain;

    rates_sp = rates_sp + QuatToDcmZ( InvertQuat(q) ) .* yaw_sp_move_rate;

    rates_sp = constrain( rates_sp, -auto_rate_max, auto_rate_max);
end

function y = constrain( x, x_min, x_max )
    y = max( min(x, x_max), x_min );
end

function dcmZ = QuatToDcmZ( quat )
    a = quat(1);
    b = quat(2);
    c = quat(3);
    d = quat(4);
    dcmZ = [ 2 * (a * c + b * d);
        2 * (c * d - a * b);
        a * a - b * b - c * c + d * d ];
end

function quat = VecsToQuat( src, dst )
    cr = cross(src, dst);
    dt = dot(src, dst);
    quat = zeros(4,1);
    locEps = 1e-5; % Don't use eps as it's a reserved variable in MATLAB
    if (norm(cr) < locEps && dt < 0)
        % Handle corner cases with 180 degree rotations
        % If the two vectors are parallel, cross product is zero
        % If they point opposite, the dot product is negative
        cr = abs(src);
        if (cr(1) < cr(2))
            if (cr(1) < cr(3))
                cr = [1; 0; 0];
            else
                cr = [0; 0; 1];
            end
        else
            if (cr(2) < cr(3))
                cr = [0; 1; 0];
            else
                cr = [0; 0; 1];
            end
        end
        quat(1) = 0;
        cr = cross(src, cr);
    else
        % Normal case, do half-way quaternion solution
        quat(1) = dt + sqrt( norm(src)^2 * norm(dst)^2 );
    end
    quat(2) = cr(1);
    quat(3) = cr(2);
    quat(4) = cr(3);
    quat = MulticopterAttitudeControl.normalize( quat );
end

function quatInv = InvertQuat( quat )
    normSq = dot( quat, quat );
    quatInv = ( quat .* [1;-1;-1;-1] ./ normSq );
end

function quatOut = QuatMult( q1, q2 )
    quatOut = [ q1(1) * q2(1) - q1(2) * q2(2) - q1(3) * q2(3) - q1(4) * q2(4) ;
        q1(1) * q2(2) + q1(2) * q2(1) + q1(3) * q2(4) - q1(4) * q2(3) ;
        q1(1) * q2(3) - q1(2) * q2(4) + q1(3) * q2(1) + q1(4) * q2(2) ;
        q1(1) * q2(4) + q1(2) * q2(3) - q1(3) * q2(2) + q1(4) * q2(1) ];
end

function out = SignNoZero( in )
    out = ( 0 <= in ) - ( in < 0 );
end

== matlab function MultirotorSimPx4v1_8ContAttOnly/Attitude controller (discrete)/MATLAB Function ==
  data: q input; rates_sp output; qd input; thrust_sp input; yaw_sp_move_rate input; attitude_gain input; auto_rate_max input
function rates_sp  = control_attitude( q, qd, thrust_sp, ...
    yaw_sp_move_rate, attitude_gain, auto_rate_max )

%thrust_sp = -thrust_sp;

roll_pitch_gain = ( attitude_gain(1) + attitude_gain(2) ) / 2;
yaw_w = constrain( attitude_gain(3) / roll_pitch_gain, 0, 1 );
attitude_gain(3) = roll_pitch_gain;

q  = q  ./ norm(q);
qd = qd ./ norm(qd);

e_z   = QuatToDcmZ( q );
e_z_d = QuatToDcmZ( qd );
qd_red = VecsToQuat( e_z, e_z_d );

qd_red = QuatMult( qd_red, q );

q_mix = QuatMult( InvertQuat(qd_red), qd );
q_mix = q_mix .* SignNoZero( q_mix(1) );

q_mix(1) = constrain( q_mix(1), -1, 1 );
q_mix(4) = constrain( q_mix(4), -1, 1 );
qd = QuatMult( qd_red, ...
    [ cos( yaw_w * acos(q_mix(1)) );
    0;
    0;
    sin( yaw_w * asin(q_mix(4)) ) ] );

qe = QuatMult( InvertQuat(q), qd );

eq = 2 .* SignNoZero(qe(1)) .* qe(2:4);

rates_sp = eq .* attitude_gain;

rates_sp = rates_sp + QuatToDcmZ( InvertQuat(q) ) .* yaw_sp_move_rate;

rates_sp = constrain( rates_sp, -auto_rate_max, auto_rate_max);
end

function y = constrain( x, x_min, x_max )
    y = max( min(x, x_max), x_min );
end

function dcmZ = QuatToDcmZ( quat )
    a = quat(1);
    b = quat(2);
    c = quat(3);
    d = quat(4);
    dcmZ = [ 2 * (a * c + b * d);
        2 * (c * d - a * b);
        a * a - b * b - c * c + d * d ];
end

function quat = VecsToQuat( src, dst )
    cr = cross(src, dst);
    dt = dot(src, dst);
    quat = zeros(4,1);
    locEps = 1e-5; % Don't use eps as it's a reserved variable in MATLAB
    if (norm(cr) < locEps && dt < 0)
        % Handle corner cases with 180 degree rotations
        % If the two vectors are parallel, cross product is zero
        % If they point opposite, the dot product is negative
        cr = abs(src);
        if (cr(1) < cr(2))
            if (cr(1) < cr(3))
                cr = [1; 0; 0];
            else
                cr = [0; 0; 1];
            end
        else
            if (cr(2) < cr(3))
                cr = [0; 1; 0];
            else
                cr = [0; 0; 1];
            end
        end
        quat(1) = 0;
        cr = cross(src, cr);
    else
        % Normal case, do half-way quaternion solution
        quat(1) = dt + sqrt( norm(src)^2 * norm(dst)^2 );
    end
    quat(2) = cr(1);
    quat(3) = cr(2);
    quat(4) = cr(3);
    quat = MulticopterAttitudeControl.normalize( quat );
end

function quatInv = InvertQuat( quat )
    normSq = dot( quat, quat );
    quatInv = ( quat .* [1;-1;-1;-1] ./ normSq );
end

function quatOut = QuatMult( q1, q2 )
    quatOut = [ q1(1) * q2(1) - q1(2) * q2(2) - q1(3) * q2(3) - q1(4) * q2(4) ;
        q1(1) * q2(2) + q1(2) * q2(1) + q1(3) * q2(4) - q1(4) * q2(3) ;
        q1(1) * q2(3) - q1(2) * q2(4) + q1(3) * q2(1) + q1(4) * q2(2) ;
        q1(1) * q2(4) + q1(2) * q2(3) - q1(3) * q2(2) + q1(4) * q2(1) ];
end

function out = SignNoZero( in )
    out = ( 0 <= in ) - ( in < 0 );
end

== matlab function MultirotorSimPx4v1_8ContAttOnly/Attitude controller (discrete)/MATLAB Function1 ==
  data: rate_p input; rate_i input; rate_d input; rates input; att_control output; rates_prev_filtered output; rates_sp input size=3; thrust_sp input; rates_filtered input size=3; rates_prev_filtered input size=3; rates_int output; rates_int input size=3
function [att_control, rates_prev_filtered, rates_int] = control_attitude_rates( rate_p, rate_i, rate_d, ...
    rates, rates_sp, thrust_sp, rates_filtered, rates_prev_filtered, rates_int )

    % values
    rate_int_lim = [ 0.3; 0.3; 0.3 ];
    tpa_breakpoint_p = 1;
    tpa_breakpoint_i = 1;
    tpa_breakpoint_d = 1;
    tpa_rate_p = 0;
    tpa_rate_i = 0;
    tpa_rate_d = 0;
    dt = 1/250;
    rate_ff = zeros(3,1);
    
    rates_p_scaled = rate_p .* pid_attenuations( tpa_breakpoint_p, tpa_rate_p, thrust_sp );
    rates_i_scaled = rate_i .* pid_attenuations( tpa_breakpoint_i, tpa_rate_i, thrust_sp );
    rates_d_scaled = rate_d .* pid_attenuations( tpa_breakpoint_d, tpa_rate_d, thrust_sp );

    rates_err = rates_sp - rates;

    %rates_filtered = LowPassFilter2pVector3Apply( obj, rates );

    att_control = rates_p_scaled .* rates_err + ...
        rates_int - ...
        rates_d_scaled .* (rates_filtered - rates_prev_filtered) / dt + ...
        rate_ff .* rates_sp;

    rates_prev_filtered = rates_filtered;

    rate_i_tmp = rates_int + rates_i_scaled .* rates_err .* dt;
    
    toKeep = isfinite(rate_i_tmp) & (rate_i_tmp > -rate_int_lim) & ...
                (rate_i_tmp < rate_int_lim);
    %rates_int = zeros(3,1);
    rates_int(toKeep) = rate_i_tmp(toKeep);
    
    rates_int = constrain( rates_int, -rate_int_lim, rate_int_lim );
end

function pidAttenuationPerAxis = pid_attenuations( tpa_breakpoint, tpa_rate, thrust_sp )
    TPA_RATE_LOWER_LIMIT = 0.05;
    tpa = 1.0 - tpa_rate * (abs(thrust_sp) - tpa_breakpoint) / (1.0 - tpa_breakpoint);
    tpa = max([TPA_RATE_LOWER_LIMIT, min([1.0, tpa])]);
    pidAttenuationPerAxis = [ tpa; tpa; 1.0 ];
end

function y = constrain( x, x_min, x_max )
    y = max( min(x, x_max), x_min );
end

== matlab function MultirotorSimPx4v1_8ContAttOnly/Attitude controller (discrete)/MATLAB Function2 ==
  data: sample input; output output; delay_element_1 input size=3; delay_element_2 input size=3; delay_element_1 output; delay_element_2 output
function [output, delay_element_1, delay_element_2]  = LowPassFilter2pVector3( sample, delay_element_1, delay_element_2 )
    sample_freq = 250;
    cutoff_freq = 30;
    [a1, a2, b0, b1, b2] = init(sample_freq, cutoff_freq);
    delay_element_0 = sample - delay_element_1.*a1 - delay_element_2.*a2;
    output = delay_element_0.*b0 + delay_element_1.*b1 + delay_element_2.*b2;
    delay_element_2 = delay_element_1;
    delay_element_1 = delay_element_0;
end

function [a1, a2, b0, b1, b2] = init(sample_freq, cutoff_freq)
    fr = sample_freq / cutoff_freq;
    ohm = tan( pi / fr);
    c = 1.0 + 2.0 * cos( pi / 4.0) * ohm + ohm * ohm;

    b0 = ohm * ohm / c;
    b1 = 2.0 * b0;
    b2 = b0;

    a1 = 2.0 * (ohm * ohm - 1.0) / c;
    a2 = (1.0 - 2.0 * cos(pi / 4.0) * ohm + ohm * ohm) / c;
end

== matlab function MultirotorSimPx4v1_8ContAttOnly/Quadrotor Euler Model/Compute etaDot ==
  data: nuBody input; eta input; etaDot output
function etaDot = computeEtaDot(nuBody, eta)
%#codegen

sPhi = sin(eta(1));
cPhi = cos(eta(1));
cTheta = cos(eta(2));
tTheta = tan(eta(2));
      
WInverse = [1, sPhi*tTheta,  cPhi*tTheta;
            0, cPhi,        -sPhi;
            0, sPhi/cTheta,  cPhi/cTheta];

etaDot = WInverse*nuBody;

== matlab function MultirotorSimPx4v1_8ContAttOnly/Quadrotor Euler Model/compute VBody ==
  data: eta input; VBody output; xiDot input
function VBody = computeVBody(eta, xiDot)
%#codegen

sphi = sin(eta(1));
sTheta = sin(eta(2));
sPsi = sin(eta(3));
cPhi = cos(eta(1));
cTheta = cos(eta(2));
cPsi = cos(eta(3));

R = [ cPsi*cTheta, cPsi*sTheta*sphi-sPsi*cPhi, cPsi*sTheta*cPhi+sPsi*sphi;
	  sPsi*cTheta, sPsi*sTheta*sphi+cPsi*cPhi, sPsi*sTheta*cPhi-cPsi*sphi;
     -sTheta,      cTheta*sphi,                cTheta*cPhi+sPsi*sphi];

VBody = R'*xiDot;
